simulink model "gm_sampleModel61741_pp_47_1_sub"  (R2023b)
settings: Solver=VariableStepAuto  StartTime=0.0  StopTime=10.0  RelTol=1e-3
libraries: simulink x46, hdlsllib x1
(part 2 of 2)

== system gm_sampleModel61741_pp_47_1_sub/Subsystem/cfblk4 ==
  note: U(k)
  note: Edge
  U : Inport  OutDataTypeStr=uint8  SampleTime=1
  Delay Input1 : UnitDelay  Description=Store in Global RAM  DisableCoverage=on  InitialCondition=vinit  SampleTime=-1  HasFrameUpgradeWarning=on
  FixPt Relational Operator : RelationalOperator  Operator=>  OutDataTypeStr=fixdt(0, 8)  ZeroCross=off  InputSameDT=off
  Nonnegative : Subsystem  mask(Compare To Zero){relop=>=, OutDataTypeStr=boolean, ZeroCross=off}
      mask prompts: relop "Simulink:masks:Operator_MP"; OutDataTypeStr "Simulink:masks:OutputDataType_MP"; ZeroCross "Simulink:masks:EnableZerocrossingDetection_MP"
      mask help: Simulink:masks:CompareToZero_MD
      mask init:
      | OutDataTypeStr = 'boolean';
      | ZeroCross = 'off';
      | blkName = 'sampleModel61741_pp_47_1_sub/Subsystem/cfblk4/Nonnegative';
      | relop = '>=';
      | setValue = 'boolean';
      mask TypeOptions relop: == | ~= | < | <= | >= | >
      mask TypeOptions OutDataTypeStr: Simulink:masks:uint8 | Simulink:masks:boolean
      mask Callback ZeroCross: sl('zeroCrossEnable', gcbh);
      mask Display: disp([relop,' 0'])
  Y : Outport  SampleTime=1
  wires:
  U/1 -> Nonnegative/1(u)
  Delay Input1/1 -> FixPt Relational Operator/2
  FixPt Relational Operator/1 -> Y/1
  Nonnegative/1(y) -> FixPt Relational Operator/1, Delay Input1/1

== system gm_sampleModel61741_pp_47_1_sub/Subsystem/cfblk41 ==
  emi_189 : Inport  OutDataTypeStr=uint8  PortDimensions=1  SampleTime=1
  Action Port : Inport  Port=2  OutDataTypeStr=boolean  SampleTime=1
  cfblk41 : Abs  SampleTime=1  OutDataTypeStr=uint8  SaturateOnIntegerOverflow=off
  cfblk41_out1bypassMux : MultiPortSwitch  DataPortOrder=Zero-based contiguous  Inputs=2  zeroidx=on  OutDataTypeStr=uint8  SampleTime=1  SaturateOnIntegerOverflow=off  InputSameDT=off
  emi_190_bypass : UnitDelay  InitialCondition="fi(0,0,8,0,\"hex\",\"00\")"  SampleTime=1
  emi_190 : Outport  SampleTime=1  InitialOutput=0
  wires:
  Action Port/1 -> cfblk41_out1bypassMux/1
  emi_189/1 -> cfblk41/1
  cfblk41/1 -> cfblk41_out1bypassMux/3
  cfblk41_out1bypassMux/1 -> emi_190_bypass/1, emi_190/1
  emi_190_bypass/1 -> cfblk41_out1bypassMux/2

== system gm_sampleModel61741_pp_47_1_sub/Subsystem/cfblk45 ==
  u : Inport  OutDataTypeStr=uint8  SampleTime=1
  FixPt Constant : Constant  DisableCoverage=on  OutDataTypeStr=Inherit: Inherit via back propagation  SampleTime=-1
  FixPt Data Type Duplicate : DataTypeDuplicate  DisableCoverage=on  NumInputPorts=3
  FixPt Sum1 : Sum  OutDataTypeStr=Inherit: Inherit via back propagation  InputSameDT=on  LockScale=on
  y : Outport  SampleTime=1
  wires:
  u/1 -> FixPt Sum1/1, FixPt Data Type Duplicate/2
  FixPt Constant/1 -> FixPt Sum1/2, FixPt Data Type Duplicate/3
  FixPt Sum1/1 -> FixPt Data Type Duplicate/1, y/1

== system gm_sampleModel61741_pp_47_1_sub/Subsystem/cfblk48 ==
  emi_213 : Inport  OutDataTypeStr=uint8  PortDimensions=1  SampleTime=1
  Action Port : Inport  Port=2  OutDataTypeStr=boolean  SampleTime=1
  Reshape : Reshape
  cfblk48_out1bypassMux : MultiPortSwitch  DataPortOrder=Zero-based contiguous  Inputs=2  zeroidx=on  OutDataTypeStr=uint8  SampleTime=1  SaturateOnIntegerOverflow=off  InputSameDT=off
  emi_214_bypass : UnitDelay  InitialCondition="fi(0,0,8,0,\"hex\",\"00\")"  SampleTime=1
  emi_214 : Outport  SampleTime=1  InitialOutput=0
  wires:
  Action Port/1 -> cfblk48_out1bypassMux/1
  emi_213/1 -> Reshape/1
  Reshape/1 -> cfblk48_out1bypassMux/3
  cfblk48_out1bypassMux/1 -> emi_214_bypass/1, emi_214/1
  emi_214_bypass/1 -> cfblk48_out1bypassMux/2

== system gm_sampleModel61741_pp_47_1_sub/Subsystem/cfblk49 ==
  u : Inport  OutDataTypeStr=uint8  SampleTime=1
  FixPt Constant : Constant  DisableCoverage=on  OutDataTypeStr=Inherit: Inherit via back propagation  SampleTime=-1
  FixPt Data Type Duplicate : DataTypeDuplicate  DisableCoverage=on  NumInputPorts=3
  FixPt Sum1 : Sum  OutDataTypeStr=Inherit: Inherit via back propagation  InputSameDT=on  LockScale=on
  y : Outport  SampleTime=1
  wires:
  u/1 -> FixPt Sum1/1, FixPt Data Type Duplicate/2
  FixPt Constant/1 -> FixPt Sum1/2, FixPt Data Type Duplicate/3
  FixPt Sum1/1 -> FixPt Data Type Duplicate/1, y/1

== system gm_sampleModel61741_pp_47_1_sub/Subsystem/cfblk50_inst ==
  in1 : Inport  OutDataTypeStr=uint8  SampleTime=1
  in2 : Inport  Port=2  OutDataTypeStr=uint8  SampleTime=1
  mul_cfblk50_dotp_mulcomp : Product  Inputs=**  OutDataTypeStr=uint8  SampleTime=1
  out1 : Outport  OutDataTypeStr=uint8  SampleTime=1
  wires:
  in1/1 -> mul_cfblk50_dotp_mulcomp/1
  in2/1 -> mul_cfblk50_dotp_mulcomp/2
  mul_cfblk50_dotp_mulcomp/1 -> out1/1

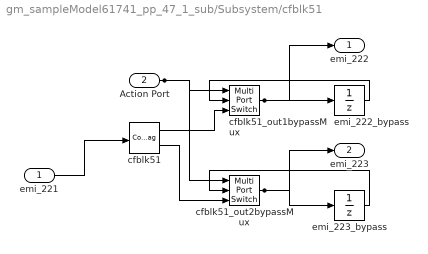
== system gm_sampleModel61741_pp_47_1_sub/Subsystem/cfblk51 ==
  emi_221 : Inport  OutDataTypeStr=uint8  PortDimensions=1  SampleTime=1
  Action Port : Inport  Port=2  OutDataTypeStr=boolean  SampleTime=1
  cfblk51 : ComplexToRealImag  SampleTime=1
  cfblk51_out1bypassMux : MultiPortSwitch  DataPortOrder=Zero-based contiguous  Inputs=2  zeroidx=on  OutDataTypeStr=uint8  SampleTime=1  SaturateOnIntegerOverflow=off  InputSameDT=off
  cfblk51_out2bypassMux : MultiPortSwitch  DataPortOrder=Zero-based contiguous  Inputs=2  zeroidx=on  OutDataTypeStr=uint8  SampleTime=1  SaturateOnIntegerOverflow=off  InputSameDT=off
  emi_222_bypass : UnitDelay  InitialCondition="fi(0,0,8,0,\"hex\",\"00\")"  SampleTime=1
  emi_223_bypass : UnitDelay  InitialCondition="fi(0,0,8,0,\"hex\",\"00\")"  SampleTime=1
  emi_222 : Outport  SampleTime=1  InitialOutput=0
  emi_223 : Outport  Port=2  SampleTime=1  InitialOutput=0
  wires:
  Action Port/1 -> cfblk51_out2bypassMux/1, cfblk51_out1bypassMux/1
  emi_221/1 -> cfblk51/1
  cfblk51/1 -> cfblk51_out1bypassMux/3
  cfblk51/2 -> cfblk51_out2bypassMux/3
  cfblk51_out1bypassMux/1 -> emi_222_bypass/1, emi_222/1
  emi_222_bypass/1 -> cfblk51_out1bypassMux/2
  cfblk51_out2bypassMux/1 -> emi_223_bypass/1, emi_223/1
  emi_223_bypass/1 -> cfblk51_out2bypassMux/2

== system gm_sampleModel61741_pp_47_1_sub/Subsystem/cfblk55 ==
  emi_238 : Inport  OutDataTypeStr=uint8  PortDimensions=1  SampleTime=1
  Action Port : Inport  Port=2  OutDataTypeStr=boolean  SampleTime=1
  cfblk55 : ComplexToRealImag  SampleTime=1
  cfblk55_out1bypassMux : MultiPortSwitch  DataPortOrder=Zero-based contiguous  Inputs=2  zeroidx=on  OutDataTypeStr=uint8  SampleTime=1  SaturateOnIntegerOverflow=off  InputSameDT=off
  cfblk55_term1 : Terminator
  emi_239_bypass : UnitDelay  InitialCondition="fi(0,0,8,0,\"hex\",\"00\")"  SampleTime=1
  emi_239 : Outport  SampleTime=1  InitialOutput=0
  wires:
  Action Port/1 -> cfblk55_out1bypassMux/1
  emi_238/1 -> cfblk55/1
  cfblk55/1 -> cfblk55_out1bypassMux/3
  cfblk55/2 -> cfblk55_term1/1
  cfblk55_out1bypassMux/1 -> emi_239_bypass/1, emi_239/1
  emi_239_bypass/1 -> cfblk55_out1bypassMux/2

== system gm_sampleModel61741_pp_47_1_sub/Subsystem/cfblk56 ==
  emi_247 : Inport  OutDataTypeStr=uint8  PortDimensions=1  SampleTime=1
  Action Port : Inport  Port=2  OutDataTypeStr=boolean  SampleTime=1
  Reshape : Reshape
  cfblk56_out1bypassMux : MultiPortSwitch  DataPortOrder=Zero-based contiguous  Inputs=2  zeroidx=on  OutDataTypeStr=uint8  SampleTime=1  SaturateOnIntegerOverflow=off  InputSameDT=off
  emi_248_bypass : UnitDelay  InitialCondition="fi(0,0,8,0,\"hex\",\"00\")"  SampleTime=1
  emi_248 : Outport  SampleTime=1  InitialOutput=0
  wires:
  Action Port/1 -> cfblk56_out1bypassMux/1
  emi_247/1 -> Reshape/1
  Reshape/1 -> cfblk56_out1bypassMux/3
  cfblk56_out1bypassMux/1 -> emi_248_bypass/1, emi_248/1
  emi_248_bypass/1 -> cfblk56_out1bypassMux/2

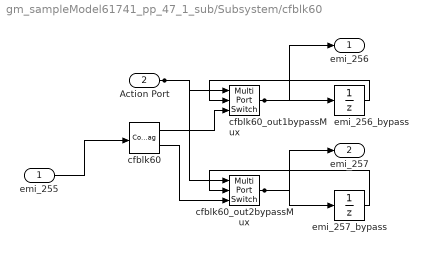
== system gm_sampleModel61741_pp_47_1_sub/Subsystem/cfblk60 ==
  emi_255 : Inport  OutDataTypeStr=uint8  PortDimensions=1  SampleTime=1
  Action Port : Inport  Port=2  OutDataTypeStr=boolean  SampleTime=1
  cfblk60 : ComplexToRealImag  SampleTime=1
  cfblk60_out1bypassMux : MultiPortSwitch  DataPortOrder=Zero-based contiguous  Inputs=2  zeroidx=on  OutDataTypeStr=uint8  SampleTime=1  SaturateOnIntegerOverflow=off  InputSameDT=off
  cfblk60_out2bypassMux : MultiPortSwitch  DataPortOrder=Zero-based contiguous  Inputs=2  zeroidx=on  OutDataTypeStr=uint8  SampleTime=1  SaturateOnIntegerOverflow=off  InputSameDT=off
  emi_256_bypass : UnitDelay  InitialCondition="fi(0,0,8,0,\"hex\",\"00\")"  SampleTime=1
  emi_257_bypass : UnitDelay  InitialCondition="fi(0,0,8,0,\"hex\",\"00\")"  SampleTime=1
  emi_256 : Outport  SampleTime=1  InitialOutput=0
  emi_257 : Outport  Port=2  SampleTime=1  InitialOutput=0
  wires:
  Action Port/1 -> cfblk60_out2bypassMux/1, cfblk60_out1bypassMux/1
  emi_255/1 -> cfblk60/1
  cfblk60/1 -> cfblk60_out1bypassMux/3
  cfblk60/2 -> cfblk60_out2bypassMux/3
  cfblk60_out1bypassMux/1 -> emi_256_bypass/1, emi_256/1
  emi_256_bypass/1 -> cfblk60_out1bypassMux/2
  cfblk60_out2bypassMux/1 -> emi_257_bypass/1, emi_257/1
  emi_257_bypass/1 -> cfblk60_out2bypassMux/2

== system gm_sampleModel61741_pp_47_1_sub/Subsystem/cfblk62 ==
  emi_264 : Inport  OutDataTypeStr=uint8  PortDimensions=1  SampleTime=1
  Action Port : Inport  Port=2  OutDataTypeStr=boolean  SampleTime=1
  cfblk62 : Signum  SampleTime=1
  cfblk62_out1bypassMux : MultiPortSwitch  DataPortOrder=Zero-based contiguous  Inputs=2  zeroidx=on  OutDataTypeStr=uint8  SampleTime=1  SaturateOnIntegerOverflow=off  InputSameDT=off
  emi_265_bypass : UnitDelay  InitialCondition="fi(0,0,8,0,\"hex\",\"00\")"  SampleTime=1
  emi_265 : Outport  SampleTime=1  InitialOutput=0
  wires:
  Action Port/1 -> cfblk62_out1bypassMux/1
  emi_264/1 -> cfblk62/1
  cfblk62/1 -> cfblk62_out1bypassMux/3
  cfblk62_out1bypassMux/1 -> emi_265_bypass/1, emi_265/1
  emi_265_bypass/1 -> cfblk62_out1bypassMux/2

== system gm_sampleModel61741_pp_47_1_sub/Subsystem/cfblk63 ==
  u : Inport  OutDataTypeStr=uint8  SampleTime=1
  FixPt Constant : Constant  DisableCoverage=on  OutDataTypeStr=Inherit: Inherit via back propagation  SampleTime=-1
  FixPt Data Type Duplicate : DataTypeDuplicate  DisableCoverage=on  NumInputPorts=3
  FixPt Sum1 : Sum  OutDataTypeStr=Inherit: Inherit via back propagation  InputSameDT=on  LockScale=on
  y : Outport  SampleTime=1
  wires:
  u/1 -> FixPt Sum1/1, FixPt Data Type Duplicate/2
  FixPt Constant/1 -> FixPt Sum1/2, FixPt Data Type Duplicate/3
  FixPt Sum1/1 -> FixPt Data Type Duplicate/1, y/1

== system gm_sampleModel61741_pp_47_1_sub/Subsystem/cfblk64 ==
  emi_280 : Inport  OutDataTypeStr=uint8  PortDimensions=1  SampleTime=1
  Action Port : Inport  Port=2  OutDataTypeStr=boolean  SampleTime=1
  cfblk64 : Abs  SampleTime=1  OutDataTypeStr=uint8  SaturateOnIntegerOverflow=off
  cfblk64_out1bypassMux : MultiPortSwitch  DataPortOrder=Zero-based contiguous  Inputs=2  zeroidx=on  OutDataTypeStr=uint8  SampleTime=1  SaturateOnIntegerOverflow=off  InputSameDT=off
  emi_281_bypass : UnitDelay  InitialCondition="fi(0,0,8,0,\"hex\",\"00\")"  SampleTime=1
  emi_281 : Outport  SampleTime=1  InitialOutput=0
  wires:
  Action Port/1 -> cfblk64_out1bypassMux/1
  emi_280/1 -> cfblk64/1
  cfblk64/1 -> cfblk64_out1bypassMux/3
  cfblk64_out1bypassMux/1 -> emi_281_bypass/1, emi_281/1
  emi_281_bypass/1 -> cfblk64_out1bypassMux/2

== system gm_sampleModel61741_pp_47_1_sub/Subsystem/cfblk65 ==
  emi_288 : Inport  OutDataTypeStr=uint8  PortDimensions=1  SampleTime=1
  Action Port : Inport  Port=2  OutDataTypeStr=boolean  SampleTime=1
  cfblk65 : Subsystem  mask(Real World Value Increment){}
      mask help: Simulink:masks:RealWorldValueIncrement_MD
      mask Display: disp('V++')
  cfblk65_out1bypassMux : MultiPortSwitch  DataPortOrder=Zero-based contiguous  Inputs=2  zeroidx=on  OutDataTypeStr=uint8  SampleTime=1  SaturateOnIntegerOverflow=off  InputSameDT=off
  emi_289_bypass : UnitDelay  InitialCondition="fi(0,0,8,0,\"hex\",\"00\")"  SampleTime=1
  emi_289 : Outport  SampleTime=1  InitialOutput=0
  wires:
  Action Port/1 -> cfblk65_out1bypassMux/1
  emi_288/1 -> cfblk65/1(u)
  cfblk65/1(y) -> cfblk65_out1bypassMux/3
  cfblk65_out1bypassMux/1 -> emi_289_bypass/1, emi_289/1
  emi_289_bypass/1 -> cfblk65_out1bypassMux/2

== system gm_sampleModel61741_pp_47_1_sub/Subsystem/cfblk66 ==
  emi_197 : Inport  OutDataTypeStr=uint8  PortDimensions=1  SampleTime=1
  Action Port : Inport  Port=2  OutDataTypeStr=boolean  SampleTime=1
  cfblk66 : Subsystem  mask(Real World Value Increment){}
      mask help: Simulink:masks:RealWorldValueIncrement_MD
      mask Display: disp('V++')
  cfblk66_out1bypassMux : MultiPortSwitch  DataPortOrder=Zero-based contiguous  Inputs=2  zeroidx=on  OutDataTypeStr=uint8  SampleTime=1  SaturateOnIntegerOverflow=off  InputSameDT=off
  emi_198_bypass : UnitDelay  InitialCondition="fi(0,0,8,0,\"hex\",\"00\")"  SampleTime=1
  emi_198 : Outport  SampleTime=1  InitialOutput=0
  wires:
  Action Port/1 -> cfblk66_out1bypassMux/1
  emi_197/1 -> cfblk66/1(u)
  cfblk66/1(y) -> cfblk66_out1bypassMux/3
  cfblk66_out1bypassMux/1 -> emi_198_bypass/1, emi_198/1
  emi_198_bypass/1 -> cfblk66_out1bypassMux/2

== system gm_sampleModel61741_pp_47_1_sub/Subsystem/cfblk71 ==
  emi_304 : Inport  OutDataTypeStr=uint8  PortDimensions=1  SampleTime=1
  Action Port : Inport  Port=2  OutDataTypeStr=boolean  SampleTime=1
  cfblk71 : MinMax
  cfblk71_out1bypassMux : MultiPortSwitch  DataPortOrder=Zero-based contiguous  Inputs=2  zeroidx=on  OutDataTypeStr=uint8  SampleTime=1  SaturateOnIntegerOverflow=off  InputSameDT=off
  emi_305_bypass : UnitDelay  InitialCondition="fi(0,0,8,0,\"hex\",\"00\")"  SampleTime=1
  emi_305 : Outport  SampleTime=1  InitialOutput=0
  wires:
  Action Port/1 -> cfblk71_out1bypassMux/1
  emi_304/1 -> cfblk71/1
  cfblk71/1 -> cfblk71_out1bypassMux/3
  cfblk71_out1bypassMux/1 -> emi_305_bypass/1, emi_305/1
  emi_305_bypass/1 -> cfblk71_out1bypassMux/2

== system gm_sampleModel61741_pp_47_1_sub/Subsystem/cfblk75 ==
  u : Inport  OutDataTypeStr=uint8  SampleTime=1
  FixPt Constant : Constant  DisableCoverage=on  OutDataTypeStr=Inherit: Inherit via back propagation  SampleTime=-1
  FixPt Data Type Duplicate : DataTypeDuplicate  DisableCoverage=on  NumInputPorts=3
  FixPt Sum1 : Sum  OutDataTypeStr=Inherit: Inherit via back propagation  InputSameDT=on  LockScale=on
  y : Outport  SampleTime=1
  wires:
  u/1 -> FixPt Sum1/1, FixPt Data Type Duplicate/2
  FixPt Constant/1 -> FixPt Sum1/2, FixPt Data Type Duplicate/3
  FixPt Sum1/1 -> FixPt Data Type Duplicate/1, y/1

== system gm_sampleModel61741_pp_47_1_sub/Subsystem/cfblk76 ==
  emi_312 : Inport  OutDataTypeStr=uint8  PortDimensions=1  SampleTime=1
  Action Port : Inport  Port=2  OutDataTypeStr=boolean  SampleTime=1
  cfblk76 : Abs  SampleTime=1  OutDataTypeStr=uint8  SaturateOnIntegerOverflow=off
  cfblk76_out1bypassMux : MultiPortSwitch  DataPortOrder=Zero-based contiguous  Inputs=2  zeroidx=on  OutDataTypeStr=uint8  SampleTime=1  SaturateOnIntegerOverflow=off  InputSameDT=off
  emi_313_bypass : UnitDelay  InitialCondition="fi(0,0,8,0,\"hex\",\"00\")"  SampleTime=1
  emi_313 : Outport  SampleTime=1  InitialOutput=0
  wires:
  Action Port/1 -> cfblk76_out1bypassMux/1
  emi_312/1 -> cfblk76/1
  cfblk76/1 -> cfblk76_out1bypassMux/3
  cfblk76_out1bypassMux/1 -> emi_313_bypass/1, emi_313/1
  emi_313_bypass/1 -> cfblk76_out1bypassMux/2

== system gm_sampleModel61741_pp_47_1_sub/Subsystem/cfblk77 ==
  emi_26 : Inport  OutDataTypeStr=uint8  PortDimensions=1  SampleTime=1
  Action Port : Inport  Port=2  OutDataTypeStr=boolean  SampleTime=1
  Reshape : Reshape
  cfblk77_out1bypassMux : MultiPortSwitch  DataPortOrder=Zero-based contiguous  Inputs=2  zeroidx=on  OutDataTypeStr=uint8  SampleTime=1  SaturateOnIntegerOverflow=off  InputSameDT=off
  emi_27_bypass : UnitDelay  InitialCondition="fi(0,0,8,0,\"hex\",\"00\")"  SampleTime=1
  emi_27 : Outport  SampleTime=1  InitialOutput=0
  wires:
  Action Port/1 -> cfblk77_out1bypassMux/1
  emi_26/1 -> Reshape/1
  Reshape/1 -> cfblk77_out1bypassMux/3
  cfblk77_out1bypassMux/1 -> emi_27_bypass/1, emi_27/1
  emi_27_bypass/1 -> cfblk77_out1bypassMux/2

== system gm_sampleModel61741_pp_47_1_sub/Subsystem/cfblk78 ==
  emi_320 : Inport  OutDataTypeStr=uint8  PortDimensions=1  SampleTime=1
  Action Port : Inport  Port=2  OutDataTypeStr=boolean  SampleTime=1
  cfblk78 : Subsystem  mask(Real World Value Increment){}
      mask help: Simulink:masks:RealWorldValueIncrement_MD
      mask Display: disp('V++')
  cfblk78_out1bypassMux : MultiPortSwitch  DataPortOrder=Zero-based contiguous  Inputs=2  zeroidx=on  OutDataTypeStr=uint8  SampleTime=1  SaturateOnIntegerOverflow=off  InputSameDT=off
  emi_321_bypass : UnitDelay  InitialCondition="fi(0,0,8,0,\"hex\",\"00\")"  SampleTime=1
  emi_321 : Outport  SampleTime=1  InitialOutput=0
  wires:
  Action Port/1 -> cfblk78_out1bypassMux/1
  emi_320/1 -> cfblk78/1(u)
  cfblk78/1(y) -> cfblk78_out1bypassMux/3
  cfblk78_out1bypassMux/1 -> emi_321_bypass/1, emi_321/1
  emi_321_bypass/1 -> cfblk78_out1bypassMux/2

== system gm_sampleModel61741_pp_47_1_sub/Subsystem/cfblk8 ==
  emi_328 : Inport  OutDataTypeStr=uint8  PortDimensions=1  SampleTime=1
  Action Port : Inport  Port=2  OutDataTypeStr=boolean  SampleTime=1
  cfblk8 : Sum  Inputs=+
  cfblk8_out1bypassMux : MultiPortSwitch  DataPortOrder=Zero-based contiguous  Inputs=2  zeroidx=on  OutDataTypeStr=uint8  SampleTime=1  SaturateOnIntegerOverflow=off  InputSameDT=off
  emi_329_bypass : UnitDelay  InitialCondition="fi(0,0,8,0,\"hex\",\"00\")"  SampleTime=1
  emi_329 : Outport  SampleTime=1  InitialOutput=0
  wires:
  Action Port/1 -> cfblk8_out1bypassMux/1
  emi_328/1 -> cfblk8/1
  cfblk8/1 -> cfblk8_out1bypassMux/3
  cfblk8_out1bypassMux/1 -> emi_329_bypass/1, emi_329/1
  emi_329_bypass/1 -> cfblk8_out1bypassMux/2

== system gm_sampleModel61741_pp_47_1_sub/Subsystem/cfblk81 ==
  emi_58 : Inport  OutDataTypeStr=uint8  PortDimensions=1  SampleTime=1
  Action Port : Inport  Port=2  OutDataTypeStr=boolean  SampleTime=1
  cfblk81 : MinMax
  cfblk81_out1bypassMux : MultiPortSwitch  DataPortOrder=Zero-based contiguous  Inputs=2  zeroidx=on  OutDataTypeStr=uint8  SampleTime=1  SaturateOnIntegerOverflow=off  InputSameDT=off
  emi_59_bypass : UnitDelay  InitialCondition="fi(0,0,8,0,\"hex\",\"00\")"  SampleTime=1
  emi_59 : Outport  SampleTime=1  InitialOutput=0
  wires:
  Action Port/1 -> cfblk81_out1bypassMux/1
  emi_58/1 -> cfblk81/1
  cfblk81/1 -> cfblk81_out1bypassMux/3
  cfblk81_out1bypassMux/1 -> emi_59_bypass/1, emi_59/1
  emi_59_bypass/1 -> cfblk81_out1bypassMux/2

== system gm_sampleModel61741_pp_47_1_sub/Subsystem/cfblk82 ==
  emi_336 : Inport  OutDataTypeStr=uint8  PortDimensions=1  SampleTime=1
  Action Port : Inport  Port=2  OutDataTypeStr=boolean  SampleTime=1
  cfblk82 : Subsystem  mask(Real World Value Increment){}
      mask help: Simulink:masks:RealWorldValueIncrement_MD
      mask Display: disp('V++')
  cfblk82_out1bypassMux : MultiPortSwitch  DataPortOrder=Zero-based contiguous  Inputs=2  zeroidx=on  OutDataTypeStr=uint8  SampleTime=1  SaturateOnIntegerOverflow=off  InputSameDT=off
  emi_337_bypass : UnitDelay  InitialCondition="fi(0,0,8,0,\"hex\",\"00\")"  SampleTime=1
  emi_337 : Outport  SampleTime=1  InitialOutput=0
  wires:
  Action Port/1 -> cfblk82_out1bypassMux/1
  emi_336/1 -> cfblk82/1(u)
  cfblk82/1(y) -> cfblk82_out1bypassMux/3
  cfblk82_out1bypassMux/1 -> emi_337_bypass/1, emi_337/1
  emi_337_bypass/1 -> cfblk82_out1bypassMux/2

== system gm_sampleModel61741_pp_47_1_sub/Subsystem/cfblk83_inst ==
  in1 : Inport  OutDataTypeStr=uint8  SampleTime=1
  in2 : Inport  Port=2  OutDataTypeStr=uint8  SampleTime=1
  mul_cfblk83_dotp_mulcomp : Product  Inputs=**  OutDataTypeStr=uint8  SampleTime=1
  out1 : Outport  OutDataTypeStr=uint8  SampleTime=1
  wires:
  in1/1 -> mul_cfblk83_dotp_mulcomp/1
  in2/1 -> mul_cfblk83_dotp_mulcomp/2
  mul_cfblk83_dotp_mulcomp/1 -> out1/1

== system gm_sampleModel61741_pp_47_1_sub/Subsystem/cfblk87 ==
  emi_344 : Inport  OutDataTypeStr=uint8  PortDimensions=1  SampleTime=1
  Action Port : Inport  Port=2  OutDataTypeStr=boolean  SampleTime=1
  cfblk87 : Subsystem  mask(Real World Value Increment){}
      mask help: Simulink:masks:RealWorldValueIncrement_MD
      mask Display: disp('V++')
  cfblk87_out1bypassMux : MultiPortSwitch  DataPortOrder=Zero-based contiguous  Inputs=2  zeroidx=on  OutDataTypeStr=uint8  SampleTime=1  SaturateOnIntegerOverflow=off  InputSameDT=off
  emi_345_bypass : UnitDelay  InitialCondition="fi(0,0,8,0,\"hex\",\"00\")"  SampleTime=1
  emi_345 : Outport  SampleTime=1  InitialOutput=0
  wires:
  Action Port/1 -> cfblk87_out1bypassMux/1
  emi_344/1 -> cfblk87/1(u)
  cfblk87/1(y) -> cfblk87_out1bypassMux/3
  cfblk87_out1bypassMux/1 -> emi_345_bypass/1, emi_345/1
  emi_345_bypass/1 -> cfblk87_out1bypassMux/2

== system gm_sampleModel61741_pp_47_1_sub/Subsystem/cfblk96_inst ==
  in1 : Inport  OutDataTypeStr=uint8  SampleTime=1
  in2 : Inport  Port=2  OutDataTypeStr=uint8  SampleTime=1
  mul_cfblk96_dotp_mulcomp : Product  Inputs=**  OutDataTypeStr=uint8  SampleTime=1
  out1 : Outport  OutDataTypeStr=uint8  SampleTime=1
  wires:
  in1/1 -> mul_cfblk96_dotp_mulcomp/1
  in2/1 -> mul_cfblk96_dotp_mulcomp/2
  mul_cfblk96_dotp_mulcomp/1 -> out1/1

== system gm_sampleModel61741_pp_47_1_sub/Subsystem/cfblk98 ==
  emi_139 : Inport  OutDataTypeStr=uint8  PortDimensions=1  SampleTime=1
  Action Port : Inport  Port=2  OutDataTypeStr=boolean  SampleTime=1
  cfblk98 : Sum  Inputs=+
  cfblk98_out1bypassMux : MultiPortSwitch  DataPortOrder=Zero-based contiguous  Inputs=2  zeroidx=on  OutDataTypeStr=uint8  SampleTime=1  SaturateOnIntegerOverflow=off  InputSameDT=off
  emi_140_bypass : UnitDelay  InitialCondition="fi(0,0,8,0,\"hex\",\"00\")"  SampleTime=1
  emi_140 : Outport  SampleTime=1  InitialOutput=0
  wires:
  Action Port/1 -> cfblk98_out1bypassMux/1
  emi_139/1 -> cfblk98/1
  cfblk98/1 -> cfblk98_out1bypassMux/3
  cfblk98_out1bypassMux/1 -> emi_140_bypass/1, emi_140/1
  emi_140_bypass/1 -> cfblk98_out1bypassMux/2

== system gm_sampleModel61741_pp_47_1_sub/Subsystem/cfblk154/cfblk154 ==
  In1 : Inport  OutDataTypeStr=uint8  PortDimensions=1  SampleTime=1
  Out1 : Outport  SampleTime=1  InitialOutput=0
  wires:
  In1/1 -> Out1/1

== system gm_sampleModel61741_pp_47_1_sub/Subsystem/cfblk172/cfblk172 ==
  in0 : Inport  OutDataTypeStr=uint8  SampleTime=1
  Action Port_out2 : EnablePort  OutDataTypeStr=boolean
  cfblk172 : Delay  DelayLength=double(2)  InitialCondition=0
  out0 : Outport  OutDataTypeStr=uint8  SampleTime=1  InitialOutput=0
  wires:
  cfblk172/1 -> out0/1
  in0/1 -> cfblk172/1

== system gm_sampleModel61741_pp_47_1_sub/Subsystem/cfblk4/Nonnegative ==
  u : Inport  OutDataTypeStr=uint8  SampleTime=1
  Compare : RelationalOperator  OutDataTypeStr=boolean  ZeroCross=off
  Constant : Constant  DisableCoverage=on  Value=0  OutDataTypeStr=Inherit: Inherit via back propagation  SampleTime=-1  PreserveConstantTs=on
  y : Outport  SampleTime=1
  wires:
  u/1 -> Compare/1
  Compare/1 -> y/1
  Constant/1 -> Compare/2

== system gm_sampleModel61741_pp_47_1_sub/Subsystem/cfblk65/cfblk65 ==
  u : Inport  OutDataTypeStr=uint8  SampleTime=1
  FixPt Constant : Constant  DisableCoverage=on  OutDataTypeStr=Inherit: Inherit via back propagation  SampleTime=-1
  FixPt Data Type Duplicate : DataTypeDuplicate  DisableCoverage=on  NumInputPorts=3
  FixPt Sum1 : Sum  OutDataTypeStr=Inherit: Inherit via back propagation  InputSameDT=on  LockScale=on
  y : Outport  SampleTime=1  InitialOutput=0
  wires:
  u/1 -> FixPt Sum1/1, FixPt Data Type Duplicate/2
  FixPt Constant/1 -> FixPt Sum1/2, FixPt Data Type Duplicate/3
  FixPt Sum1/1 -> FixPt Data Type Duplicate/1, y/1

== system gm_sampleModel61741_pp_47_1_sub/Subsystem/cfblk66/cfblk66 ==
  u : Inport  OutDataTypeStr=uint8  SampleTime=1
  FixPt Constant : Constant  DisableCoverage=on  OutDataTypeStr=Inherit: Inherit via back propagation  SampleTime=-1
  FixPt Data Type Duplicate : DataTypeDuplicate  DisableCoverage=on  NumInputPorts=3
  FixPt Sum1 : Sum  OutDataTypeStr=Inherit: Inherit via back propagation  InputSameDT=on  LockScale=on
  y : Outport  SampleTime=1  InitialOutput=0
  wires:
  u/1 -> FixPt Sum1/1, FixPt Data Type Duplicate/2
  FixPt Constant/1 -> FixPt Sum1/2, FixPt Data Type Duplicate/3
  FixPt Sum1/1 -> FixPt Data Type Duplicate/1, y/1

== system gm_sampleModel61741_pp_47_1_sub/Subsystem/cfblk78/cfblk78 ==
  u : Inport  OutDataTypeStr=uint8  SampleTime=1
  FixPt Constant : Constant  DisableCoverage=on  OutDataTypeStr=Inherit: Inherit via back propagation  SampleTime=-1
  FixPt Data Type Duplicate : DataTypeDuplicate  DisableCoverage=on  NumInputPorts=3
  FixPt Sum1 : Sum  OutDataTypeStr=Inherit: Inherit via back propagation  InputSameDT=on  LockScale=on
  y : Outport  SampleTime=1  InitialOutput=0
  wires:
  u/1 -> FixPt Sum1/1, FixPt Data Type Duplicate/2
  FixPt Constant/1 -> FixPt Sum1/2, FixPt Data Type Duplicate/3
  FixPt Sum1/1 -> FixPt Data Type Duplicate/1, y/1

== system gm_sampleModel61741_pp_47_1_sub/Subsystem/cfblk82/cfblk82 ==
  u : Inport  OutDataTypeStr=uint8  SampleTime=1
  FixPt Constant : Constant  DisableCoverage=on  OutDataTypeStr=Inherit: Inherit via back propagation  SampleTime=-1
  FixPt Data Type Duplicate : DataTypeDuplicate  DisableCoverage=on  NumInputPorts=3
  FixPt Sum1 : Sum  OutDataTypeStr=Inherit: Inherit via back propagation  InputSameDT=on  LockScale=on
  y : Outport  SampleTime=1  InitialOutput=0
  wires:
  u/1 -> FixPt Sum1/1, FixPt Data Type Duplicate/2
  FixPt Constant/1 -> FixPt Sum1/2, FixPt Data Type Duplicate/3
  FixPt Sum1/1 -> FixPt Data Type Duplicate/1, y/1

== system gm_sampleModel61741_pp_47_1_sub/Subsystem/cfblk87/cfblk87 ==
  u : Inport  OutDataTypeStr=uint8  SampleTime=1
  FixPt Constant : Constant  DisableCoverage=on  OutDataTypeStr=Inherit: Inherit via back propagation  SampleTime=-1
  FixPt Data Type Duplicate : DataTypeDuplicate  DisableCoverage=on  NumInputPorts=3
  FixPt Sum1 : Sum  OutDataTypeStr=Inherit: Inherit via back propagation  InputSameDT=on  LockScale=on
  y : Outport  SampleTime=1  InitialOutput=0
  wires:
  u/1 -> FixPt Sum1/1, FixPt Data Type Duplicate/2
  FixPt Constant/1 -> FixPt Sum1/2, FixPt Data Type Duplicate/3
  FixPt Sum1/1 -> FixPt Data Type Duplicate/1, y/1
